simulink model "sim13_rampas"  (R2015b)
settings: Solver=VariableStepAuto  StartTime=0.0  StopTime=tt  RelTol=1e-3
values from neighbouring files (symbols this model uses):
  dy_inicial = 0    [Lab2.m]
  k1 = 1/yl    (= 10)    [Lab2.m]    (also in u_valor.m = 1/yl)
  k2 = sqrt(2*k1)    [Lab2.m]    (also in u_valor.m)
  t_rampa = 2    [Lab2.m]
  y_inicial = 1    [Lab2.m]
  yl = 0.1    [Lab2.m]
libraries: simulink x1
settings Model: Creator=Alice  LastModifiedBy=Alice

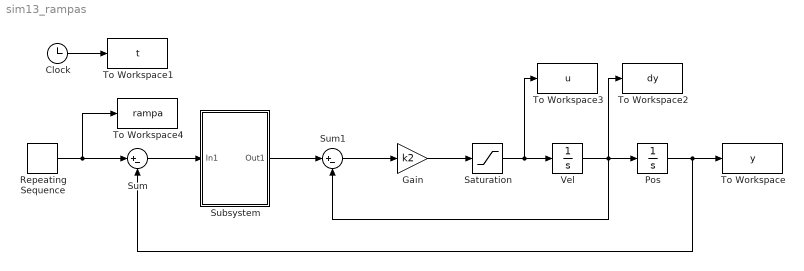
== system sim13_rampas ==
  Clock : Clock
  Gain : Gain  Gain=k2
  Pos : Integrator  InitialCondition=y_inicial
  Repeating Sequence : simulink/Sources/Repeating Sequence  rep_seq_t=[0 t_rampa]  rep_seq_y=[0 2]
  Saturation : Saturate  UpperLimit=1  LowerLimit=-1
  Subsystem : Subsystem
  Sum : Sum  Inputs=|+-
  Sum1 : Sum  Inputs=|+-
  To Workspace : ToWorkspace  VariableName=y  SampleTime=0.1
  To Workspace1 : ToWorkspace  VariableName=t  SampleTime=0.1
  To Workspace2 : ToWorkspace  VariableName=dy  SampleTime=0.1
  To Workspace3 : ToWorkspace  VariableName=u  SampleTime=0.1
  To Workspace4 : ToWorkspace  VariableName=rampa  SampleTime=-1
  Vel : Integrator  InitialCondition=dy_inicial
  wires:
  Sum/1 -> Subsystem/1(In1)
  Subsystem/1(Out1) -> Sum1/1
  Sum1/1 -> Gain/1
  Gain/1 -> Saturation/1
  Saturation/1 -> To Workspace3/1, Vel/1
  Vel/1 -> To Workspace2/1, Sum1/2, Pos/1
  Pos/1 -> To Workspace/1, Sum/2
  Clock/1 -> To Workspace1/1
  Repeating Sequence/1 -> Sum/1, To Workspace4/1

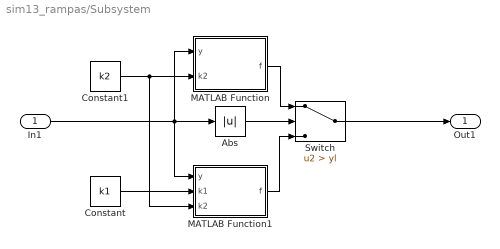
== system sim13_rampas/Subsystem ==
  In1 : Inport
  Abs : Abs
  Constant : Constant  Value=k1
  Constant1 : Constant  Value=k2
  MATLAB Function : MATLAB Function  TreatAsAtomicUnit=on
  MATLAB Function1 : MATLAB Function  TreatAsAtomicUnit=on
  Switch : Switch  Criteria=u2 > Threshold  Threshold=yl
  Out1 : Outport
  wires:
  In1/1 -> Abs/1, MATLAB Function/1(y), MATLAB Function1/1(y)
  Switch/1 -> Out1/1
  MATLAB Function/1(f) -> Switch/1
  Constant/1 -> MATLAB Function1/2(k1)
  MATLAB Function1/1(f) -> Switch/3
  Abs/1 -> Switch/2
  Constant1/1 -> MATLAB Function1/3(k2), MATLAB Function/2(k2)

== matlab function sim13_rampas/Subsystem/MATLAB Function1 ==
  data: y input; k1 input; f output; k2 input
function f = fcn(y,k1,k2)

f=(k1/k2)*(y);

end

== matlab function sim13_rampas/Subsystem/MATLAB Function ==
  data: y input; f output; k2 input
function f = fcn(y,k2)

f=sign(y)*(sqrt(2*abs(y))-(1/k2));

end
